simulink model "sldemo_foucault"  (Simulink 7.6)
settings: Solver=ode23t  StartTime=0.0  StopTime=3600  FixedStep=.1  RelTol=1e-5
InitFcn:
  | sldemo_foucault_data;
values from neighbouring files (symbols this model uses):
  g = 9.83    [sldemo_foucault_data.m]    (also in sldemo_tankgui.m = LocalDrawTank(hilim, lolim, inflow, outflow, area); sldemo_tanksfun.m = get(ax,'UserData'))
  initial_x = L/100    (= 0.67)    [sldemo_foucault_data.m]
  initial_xdot = 0    [sldemo_foucault_data.m]
  initial_y = 0    [sldemo_foucault_data.m]
  initial_ydot = 0    [sldemo_foucault_data.m]
  L = 67    [sldemo_foucault_data.m]
  lambda = 49/180*pi    (= 0.855211333477)    [sldemo_foucault_data.m]
  Omega = 2*pi/86400    (= 7.27220521664e-05)    [sldemo_foucault_data.m]
CloseFcn:
  | close(findobj('Tag','CloseMe'));
settings Model: Creator=The MathWorks Inc.
settings DataIOCC: LimitDataPoints=off  SaveFormat=StructureWithTime  SaveOutput=off  SaveTime=off  SignalLoggingName=sldemo_foucault_output
settings OptimizationCC: InitFltsAndDblsToZero=on
settings DebuggingCC: SaveWithParameterizedLinksMsg=none  SignalResolutionControl=TryResolveAllWithWarning  SolverPrmCheckMsg=none
settings GRTTargetCC: TargetFcnLib=ansi_tfl_tmw.mat

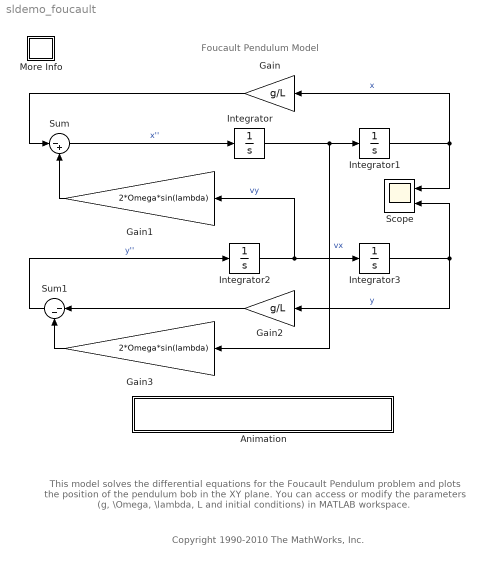
== system sldemo_foucault ==
  note: This model solves the differential equations for the Foucault Pendulum problem
      | and plots the position of the pendulum bob in the XY plane. You can access or modify
      | the parameters (g, \Omega, \lambda, L and initial conditions) in MATLAB workspace.
  note: Foucault Pendulum Model
  note: Copyright 1990-2010 The MathWorks, Inc.
  Animation : Subsystem
      settings: OpenFcn=|
      | if exist('sldemo_foucault_output','var')
      |    sldemo_foucault_animate;
      | else
      |    display('sldemo_foucault_output not found');
      |    display('Please run the simulation and then animate the results');
      | end
      mask Display: disp('Double Click Here to Animate Results')
  Gain : Gain  Gain=g/L
  Gain1 : Gain  Gain=2*Omega*sin(lambda)
  Gain2 : Gain  Gain=g/L
  Gain3 : Gain  Gain=2*Omega*sin(lambda)
  Integrator : Integrator  InitialCondition=initial_xdot
  Integrator1 : Integrator  InitialCondition=initial_x
  Integrator2 : Integrator  InitialCondition=initial_ydot
  Integrator3 : Integrator  InitialCondition=initial_y
  More Info : Subsystem
      settings: OpenFcn=showdemo(bdroot(gcs))
      mask Display: disp('?')
  Scope : Scope  NumInputPorts=2
      settings: TickLabels=on  TimeRange=4000  YMin=-0.8~-0.2  YMax=0.8~0.15  SaveName=output
  Sum : Sum  Inputs=|-+
  Sum1 : Sum  Inputs=|--
  wires:
  Integrator/1 -> Integrator1/1, Gain3/1  "vx"
  Integrator1/1 -> Scope/1, Gain/1  "x"
  Sum/1 -> Integrator/1  "x''"
  Gain/1 -> Sum/1
  Gain1/1 -> Sum/2
  Integrator2/1 -> Integrator3/1, Gain1/1  "vy"
  Gain2/1 -> Sum1/1
  Gain3/1 -> Sum1/2
  Sum1/1 -> Integrator2/1  "y''"
  Integrator3/1 -> Gain2/1, Scope/2  "y"

== system sldemo_foucault/Animation ==

== system sldemo_foucault/More Info ==
